simulink model "exp2"  (R2024b)
settings: Solver=VariableStepAuto  StartTime=0.0  StopTime=1  RelTol=1e-3
InitFcn:
  | VOC = 32.9;
  | Iscn = 8.21;
  | k = 1.38e-23;
  | NS = 54;
  | Np = 1;
  | G1 = 1000;
  | G2 = 806;
  | G3 = 506;
  | Gn = 1000;
  | Kv = -0.0123;
  | K1 = 0.0032;
  | T = 301;
  | Tn = 300;
  | q = 1.6e-19;
  | T0n = 9.58e-8;
  | Eg = 1.12;
  | Ign = 8.214;
  | Rs = 0.221;
  | Rp = 414.5;
  | a = 1.0;
libraries: spsVoltageMeasurementLib x7, spsSeriesRLCBranchLib x6, spsDiodeLib x3, spsControlledCurrentSourceLib x3, spsControlledVoltageSourceLib x1, spsCurrentMeasurementLib x1, simulink x1, spspowerguiLib x1
settings Model: Creator=91861  LastModifiedBy=palla

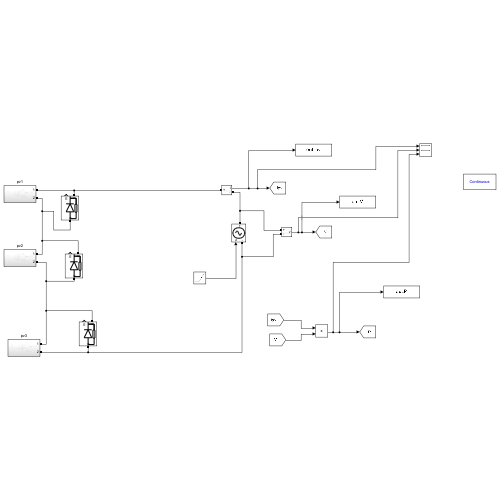
[thumbnail: Simulink's stored preview of the top-level diagram]
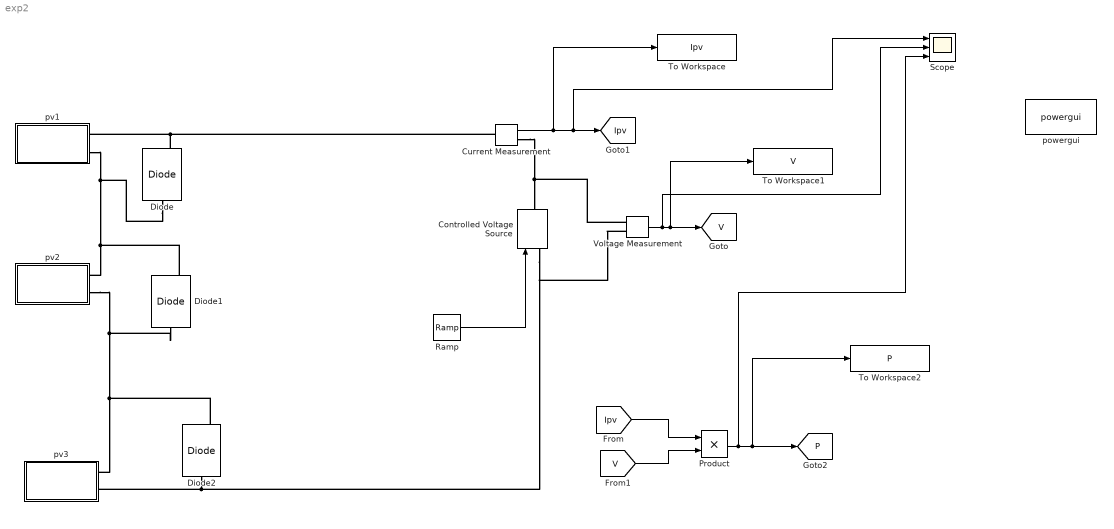
== system exp2 ==
  Controlled Voltage Source : spsControlledVoltageSourceLib/Controlled Voltage Source  Initialize=on  Source_Type=AC  Amplitude=0  Phase=0  Frequency=0  Measurements=None
  Current Measurement : spsCurrentMeasurementLib/Current Measurement  PhasorSimulation=off  OutputType=Complex  PSBequivalent=0
  Diode : spsDiodeLib/Diode  Ron=0.001  Lon=0  Vf=0.8  IC=0  UseSnubber=0  Rs=500  Cs=250e-9  Measurements=on
  Diode1 : spsDiodeLib/Diode  Ron=0.001  Lon=0  Vf=0.8  IC=0  UseSnubber=0  Rs=500  Cs=250e-9  Measurements=on
  Diode2 : spsDiodeLib/Diode  Ron=0.001  Lon=0  Vf=0.8  IC=0  UseSnubber=0  Rs=500  Cs=250e-9  Measurements=on
  Product : Product
  Ramp : simulink/Sources/Ramp  slope=100  start=0  InitialOutput=0
  Scope : Scope  NumInputPorts=3
  To Workspace : ToWorkspace  VariableName=Ipv  SampleTime=-1
  To Workspace1 : ToWorkspace  VariableName=V  SampleTime=-1
  To Workspace2 : ToWorkspace  VariableName=P  SampleTime=-1
  Voltage Measurement : spsVoltageMeasurementLib/Voltage Measurement  PhasorSimulation=off  OutputType=Complex  PSBequivalent=0
  powergui : spspowerguiLib/powergui  Priority=1  SimulationMode=Continuous  SampleTime=50e-6  frequency=60  Iterations=50  frequencyindice=0  Pbase=100e6  ErrMax=1e-4  UnitsV=kV  UnitsW=MW  buscounter=0  FunctionMessages=off  echomessages=off  EnableUseOfTLC=off  CurrentSourceSwitches=off  DisableSnubberDevices=off  DisableRonSwitches=off  DisableVfSwitches=off  DisplayEquations=off  AutomaticDiscreteSolvers=off  SolverType=Tustin/Backward Euler (TBE)  Interpol=off  ExternalGateDelay=off  methode=off  Ts=100  x0status=blocks  SPID=on  SwTol=0  HookPort=off  NonlinearTolerance=1e-4  nMaxIteration=100  ContinueOnMaxIteration=off  RestoreLinks=warning  ResistiveCurrentMeasurement=off  Frange=[0:2:500]  Ylog=off  Xlog=on  ShowGrid=off  save=off  variable=ZData  structure=0  ZoomFFT=off  StartTime=0.0  cycles=1  DisplayStyle=1  fundamental=60  FreqAxis=off  MaxFrequency=1000  frequencyindicesteady=1  RmsSteady=1  display=off
  pv1 : Subsystem
  pv2 : Subsystem
  pv3 : Subsystem
  tag scope: Ipv=global, P=global, V=global
  wires:
  Voltage Measurement/1 -> Scope/2, To Workspace1/1, [V]
  Current Measurement/1 -> To Workspace/1, Scope/1, [Ipv]
  Ramp/1 -> Controlled Voltage Source/1
  [Ipv] -> Product/1
  [V] -> Product/2
  Product/1 -> Scope/3, To Workspace2/1, [P]
  connections:
  pv1/LConn2 -- Diode/LConn1 -- Diode1/RConn1 -- pv2/LConn1
  pv2/LConn2 -- Diode1/LConn1 -- Diode2/RConn1 -- pv3/LConn1
  Diode/RConn1 -- Current Measurement/LConn1 -- pv1/LConn1
  Diode2/LConn1 -- Voltage Measurement/LConn2 -- Controlled Voltage Source/LConn1 -- pv3/LConn2
  Current Measurement/RConn1 -- Voltage Measurement/LConn1 -- Controlled Voltage Source/RConn1

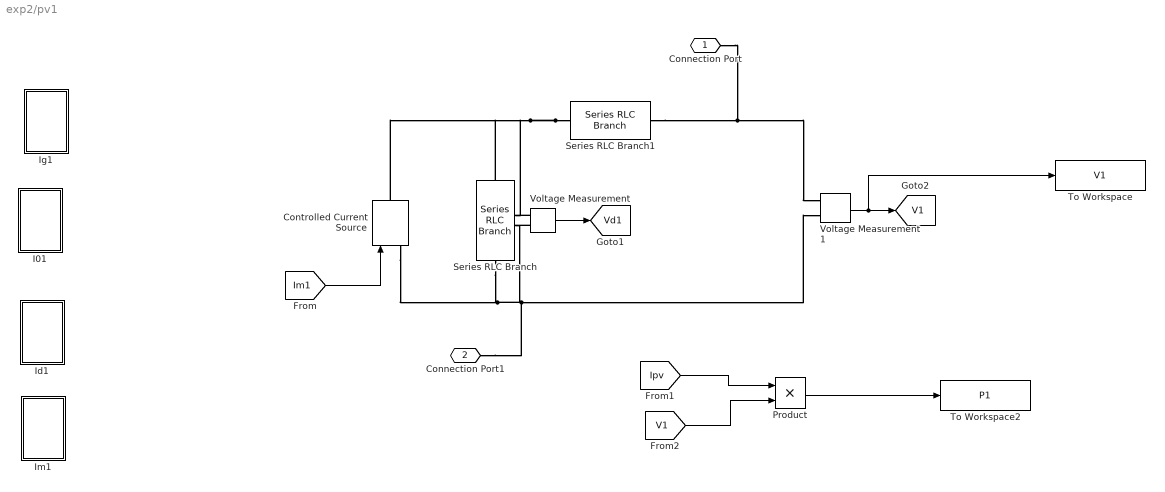
== system exp2/pv1 ==
  Controlled Current Source : spsControlledCurrentSourceLib/Controlled Current Source  Initialize=on  Source_Type=AC  Amplitude=0  Phase=0  Frequency=0  Measurements=None
  I01 : Subsystem
  Id1 : Subsystem
  Ig1 : Subsystem
  Im1 : Subsystem
  Product : Product
  Series RLC Branch : spsSeriesRLCBranchLib/Series RLC Branch  LConnTagsString=__new0  RConnTagsString=__new0  BranchType=R  Resistance=Rp  Inductance=1e-3  SetiL0=off  InitialCurrent=0  Capacitance=1e-6  Setx0=off  InitialVoltage=0  Measurements=None
  Series RLC Branch1 : spsSeriesRLCBranchLib/Series RLC Branch  LConnTagsString=__new0  RConnTagsString=__new0  BranchType=R  Resistance=Rs  Inductance=1e-3  SetiL0=off  InitialCurrent=0  Capacitance=1e-6  Setx0=off  InitialVoltage=0  Measurements=None
  To Workspace : ToWorkspace  VariableName=V1  SampleTime=-1
  To Workspace2 : ToWorkspace  VariableName=P1  SampleTime=-1
  Voltage Measurement : spsVoltageMeasurementLib/Voltage Measurement  PhasorSimulation=off  OutputType=Complex  PSBequivalent=0
  Voltage Measurement1 : spsVoltageMeasurementLib/Voltage Measurement  PhasorSimulation=off  OutputType=Complex  PSBequivalent=0
  Connection Port : PMIOPort  Side=Left
  Connection Port1 : PMIOPort  Port=2  Side=Left
  tag scope: V1=global, Vd1=global
  wires:
  Voltage Measurement1/1 -> To Workspace/1, [V1]
  [Ipv] -> Product/1
  Voltage Measurement/1 -> [Vd1]
  [V1] -> Product/2
  Product/1 -> To Workspace2/1
  [Im1] -> Controlled Current Source/1
  connections:
  Series RLC Branch1/LConn1 -- Controlled Current Source/RConn1 -- Series RLC Branch/LConn1 -- Voltage Measurement/LConn1
  Controlled Current Source/LConn1 -- Series RLC Branch/RConn1 -- Voltage Measurement/LConn2 -- Connection Port1/RConn1 -- Voltage Measurement1/LConn2
  Series RLC Branch1/RConn1 -- Connection Port/RConn1 -- Voltage Measurement1/LConn1

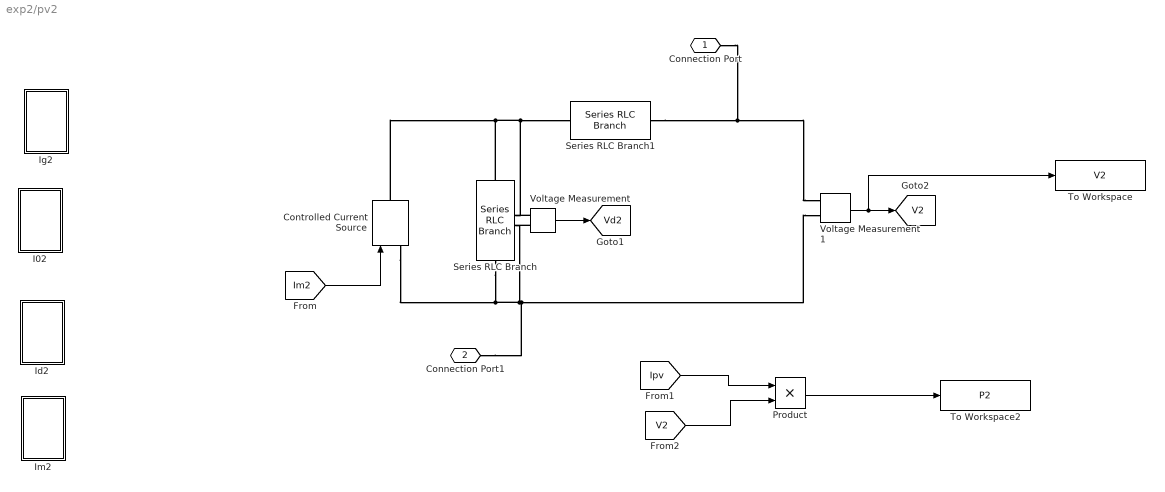
== system exp2/pv2 ==
  Controlled Current Source : spsControlledCurrentSourceLib/Controlled Current Source  Initialize=on  Source_Type=AC  Amplitude=0  Phase=0  Frequency=0  Measurements=None
  I02 : Subsystem
  Id2 : Subsystem
  Ig2 : Subsystem
  Im2 : Subsystem
  Product : Product
  Series RLC Branch : spsSeriesRLCBranchLib/Series RLC Branch  LConnTagsString=__new0  RConnTagsString=__new0  BranchType=R  Resistance=Rp  Inductance=1e-3  SetiL0=off  InitialCurrent=0  Capacitance=1e-6  Setx0=off  InitialVoltage=0  Measurements=None
  Series RLC Branch1 : spsSeriesRLCBranchLib/Series RLC Branch  LConnTagsString=__new0  RConnTagsString=__new0  BranchType=R  Resistance=Rs  Inductance=1e-3  SetiL0=off  InitialCurrent=0  Capacitance=1e-6  Setx0=off  InitialVoltage=0  Measurements=None
  To Workspace : ToWorkspace  VariableName=V2  SampleTime=-1
  To Workspace2 : ToWorkspace  VariableName=P2  SampleTime=-1
  Voltage Measurement : spsVoltageMeasurementLib/Voltage Measurement  PhasorSimulation=off  OutputType=Complex  PSBequivalent=0
  Voltage Measurement1 : spsVoltageMeasurementLib/Voltage Measurement  PhasorSimulation=off  OutputType=Complex  PSBequivalent=0
  Connection Port : PMIOPort  Side=Left
  Connection Port1 : PMIOPort  Port=2  Side=Left
  tag scope: V2=global, Vd2=global
  wires:
  Voltage Measurement1/1 -> To Workspace/1, [V2]
  [Ipv] -> Product/1
  Voltage Measurement/1 -> [Vd2]
  [V2] -> Product/2
  Product/1 -> To Workspace2/1
  [Im2] -> Controlled Current Source/1
  connections:
  Controlled Current Source/RConn1 -- Series RLC Branch/LConn1 -- Voltage Measurement/LConn1 -- Series RLC Branch1/LConn1
  Voltage Measurement1/LConn2 -- Controlled Current Source/LConn1 -- Series RLC Branch/RConn1 -- Voltage Measurement/LConn2 -- Connection Port1/RConn1
  Voltage Measurement1/LConn1 -- Series RLC Branch1/RConn1 -- Connection Port/RConn1

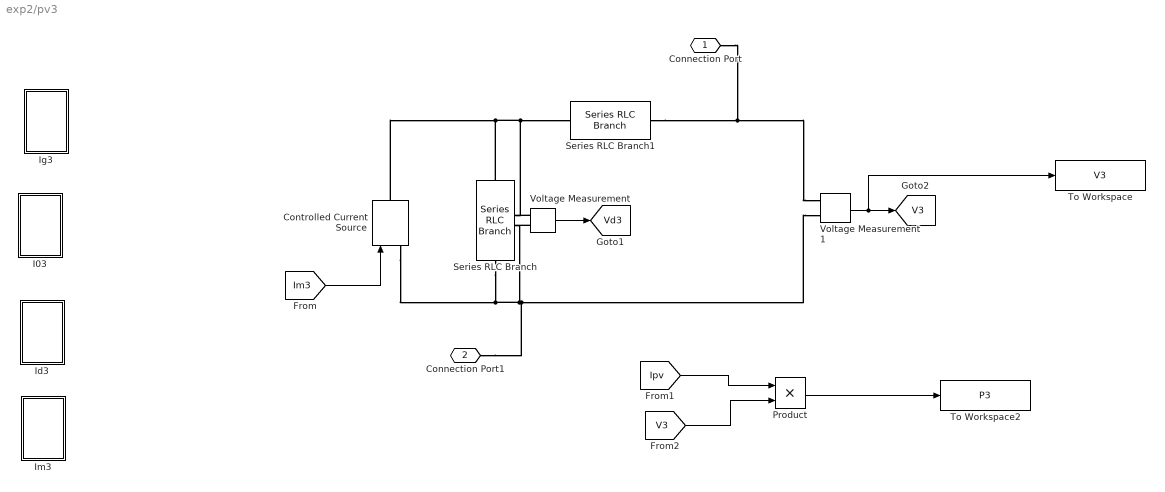
== system exp2/pv3 ==
  Controlled Current Source : spsControlledCurrentSourceLib/Controlled Current Source  Initialize=on  Source_Type=AC  Amplitude=0  Phase=0  Frequency=0  Measurements=None
  I03 : Subsystem
  Id3 : Subsystem
  Ig3 : Subsystem
  Im3 : Subsystem
  Product : Product
  Series RLC Branch : spsSeriesRLCBranchLib/Series RLC Branch  LConnTagsString=__new0  RConnTagsString=__new0  BranchType=R  Resistance=Rp  Inductance=1e-3  SetiL0=off  InitialCurrent=0  Capacitance=1e-6  Setx0=off  InitialVoltage=0  Measurements=None
  Series RLC Branch1 : spsSeriesRLCBranchLib/Series RLC Branch  LConnTagsString=__new0  RConnTagsString=__new0  BranchType=R  Resistance=Rs  Inductance=1e-3  SetiL0=off  InitialCurrent=0  Capacitance=1e-6  Setx0=off  InitialVoltage=0  Measurements=None
  To Workspace : ToWorkspace  VariableName=V3  SampleTime=-1
  To Workspace2 : ToWorkspace  VariableName=P3  SampleTime=-1
  Voltage Measurement : spsVoltageMeasurementLib/Voltage Measurement  PhasorSimulation=off  OutputType=Complex  PSBequivalent=0
  Voltage Measurement1 : spsVoltageMeasurementLib/Voltage Measurement  PhasorSimulation=off  OutputType=Complex  PSBequivalent=0
  Connection Port : PMIOPort  Side=Left
  Connection Port1 : PMIOPort  Port=2  Side=Left
  tag scope: V3=global, Vd3=global
  wires:
  Voltage Measurement1/1 -> To Workspace/1, [V3]
  [Ipv] -> Product/1
  Voltage Measurement/1 -> [Vd3]
  [V3] -> Product/2
  Product/1 -> To Workspace2/1
  [Im3] -> Controlled Current Source/1
  connections:
  Controlled Current Source/RConn1 -- Series RLC Branch/LConn1 -- Voltage Measurement/LConn1 -- Series RLC Branch1/LConn1
  Voltage Measurement1/LConn2 -- Controlled Current Source/LConn1 -- Series RLC Branch/RConn1 -- Voltage Measurement/LConn2 -- Connection Port1/RConn1
  Voltage Measurement1/LConn1 -- Series RLC Branch1/RConn1 -- Connection Port/RConn1

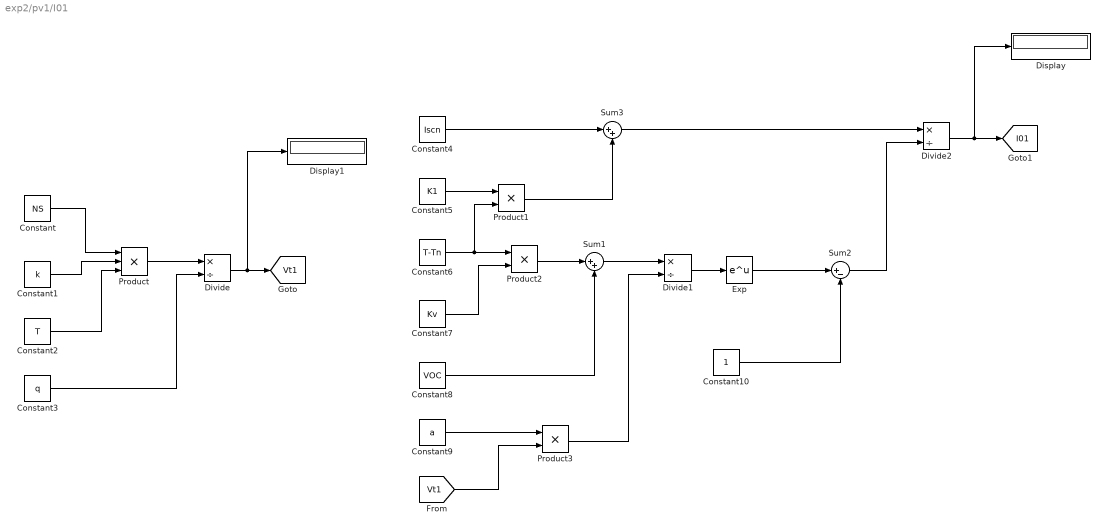
== system exp2/pv1/I01 ==
  Constant : Constant  Value=NS
  Constant1 : Constant  Value=k
  Constant10 : Constant
  Constant2 : Constant  Value=T
  Constant3 : Constant  Value=q
  Constant4 : Constant  Value=Iscn
  Constant5 : Constant  Value=K1
  Constant6 : Constant  Value=T-Tn
  Constant7 : Constant  Value=Kv
  Constant8 : Constant  Value=VOC
  Constant9 : Constant  Value=a
  Display : Display
  Display1 : Display
  Divide : Product  Inputs=*/
  Divide1 : Product  Inputs=*/
  Divide2 : Product  Inputs=*/
  Exp : Math
  Product : Product  Inputs=3
  Product1 : Product
  Product2 : Product
  Product3 : Product
  Sum1 : Sum  Inputs=|++
  Sum2 : Sum  Inputs=|+-
  Sum3 : Sum  Inputs=|++
  tag scope: I01=global, Vt1=global
  wires:
  Constant8/1 -> Sum1/2
  Product2/1 -> Sum1/1
  Constant6/1 -> Product1/2, Product2/1
  Constant5/1 -> Product1/1
  Constant/1 -> Product/1
  Divide2/1 -> Display/1, [I01]
  [Vt1] -> Product3/2
  Product1/1 -> Sum3/2
  Sum1/1 -> Divide1/1
  Sum2/1 -> Divide2/2
  Constant10/1 -> Sum2/2
  Constant7/1 -> Product2/2
  Constant1/1 -> Product/2
  Exp/1 -> Sum2/1
  Product3/1 -> Divide1/2
  Divide/1 -> Display1/1, [Vt1]
  Constant2/1 -> Product/3
  Constant3/1 -> Divide/2
  Divide1/1 -> Exp/1
  Product/1 -> Divide/1
  Constant4/1 -> Sum3/1
  Constant9/1 -> Product3/1
  Sum3/1 -> Divide2/1

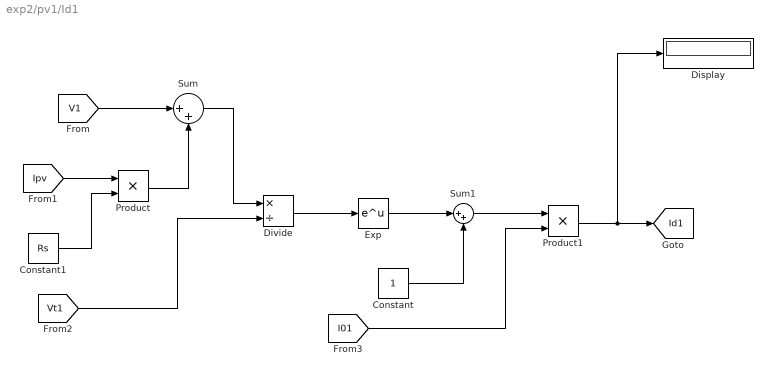
== system exp2/pv1/Id1 ==
  Constant : Constant
  Constant1 : Constant  Value=Rs
  Display : Display
  Divide : Product  Inputs=*/
  Exp : Math
  Product : Product
  Product1 : Product
  Sum : Sum  Inputs=|++
  Sum1 : Sum  Inputs=|++
  tag scope: Id1=global
  wires:
  [Ipv] -> Product/1
  [V1] -> Sum/1
  Divide/1 -> Exp/1
  [Vt1] -> Divide/2
  Sum1/1 -> Product1/1
  Product/1 -> Sum/2
  Constant1/1 -> Product/2
  Product1/1 -> Display/1, [Id1]
  Constant/1 -> Sum1/2
  [I01] -> Product1/2
  Exp/1 -> Sum1/1
  Sum/1 -> Divide/1

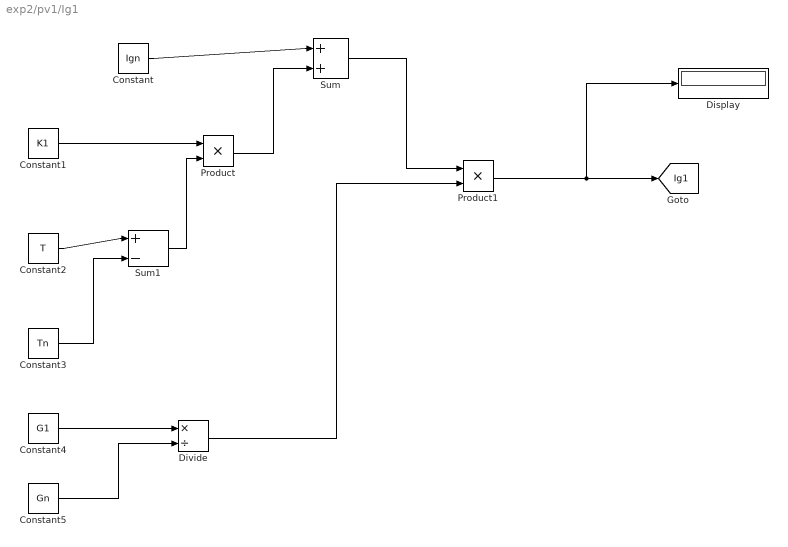
== system exp2/pv1/Ig1 ==
  Constant : Constant  Value=Ign
  Constant1 : Constant  Value=K1
  Constant2 : Constant  Value=T
  Constant3 : Constant  Value=Tn
  Constant4 : Constant  Value=G1
  Constant5 : Constant  Value=Gn
  Display : Display
  Divide : Product  Inputs=*/
  Product : Product
  Product1 : Product
  Sum : Sum  Inputs=|++
  Sum1 : Sum  Inputs=|+-
  tag scope: Ig1=global
  wires:
  Constant2/1 -> Sum1/1
  Sum/1 -> Product1/1
  Constant3/1 -> Sum1/2
  Product1/1 -> [Ig1], Display/1
  Constant/1 -> Sum/1
  Divide/1 -> Product1/2
  Sum1/1 -> Product/2
  Constant4/1 -> Divide/1
  Product/1 -> Sum/2
  Constant5/1 -> Divide/2
  Constant1/1 -> Product/1

== system exp2/pv1/Im1 ==
  Display : Display
  Sum : Sum  Inputs=|+-
  tag scope: Im1=global
  wires:
  Sum/1 -> Display/1, [Im1]
  [Ig1] -> Sum/1
  [Id1] -> Sum/2

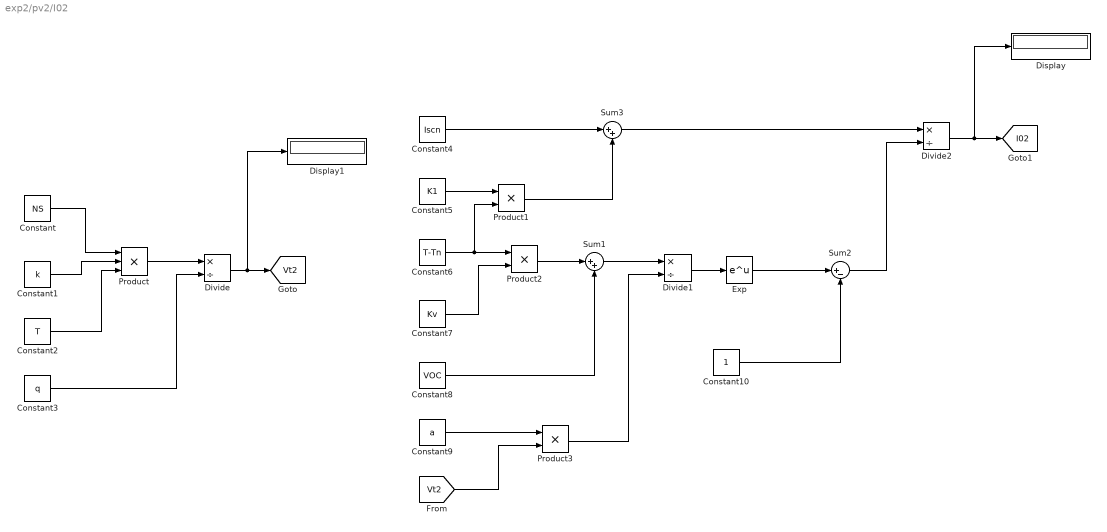
== system exp2/pv2/I02 ==
  Constant : Constant  Value=NS
  Constant1 : Constant  Value=k
  Constant10 : Constant
  Constant2 : Constant  Value=T
  Constant3 : Constant  Value=q
  Constant4 : Constant  Value=Iscn
  Constant5 : Constant  Value=K1
  Constant6 : Constant  Value=T-Tn
  Constant7 : Constant  Value=Kv
  Constant8 : Constant  Value=VOC
  Constant9 : Constant  Value=a
  Display : Display
  Display1 : Display
  Divide : Product  Inputs=*/
  Divide1 : Product  Inputs=*/
  Divide2 : Product  Inputs=*/
  Exp : Math
  Product : Product  Inputs=3
  Product1 : Product
  Product2 : Product
  Product3 : Product
  Sum1 : Sum  Inputs=|++
  Sum2 : Sum  Inputs=|+-
  Sum3 : Sum  Inputs=|++
  tag scope: I02=global, Vt2=global
  wires:
  Constant8/1 -> Sum1/2
  Product2/1 -> Sum1/1
  Constant6/1 -> Product1/2, Product2/1
  Constant5/1 -> Product1/1
  Constant/1 -> Product/1
  Divide2/1 -> Display/1, [I02]
  [Vt2] -> Product3/2
  Product1/1 -> Sum3/2
  Sum1/1 -> Divide1/1
  Sum2/1 -> Divide2/2
  Constant10/1 -> Sum2/2
  Constant7/1 -> Product2/2
  Constant1/1 -> Product/2
  Exp/1 -> Sum2/1
  Product3/1 -> Divide1/2
  Divide/1 -> Display1/1, [Vt2]
  Constant2/1 -> Product/3
  Constant3/1 -> Divide/2
  Divide1/1 -> Exp/1
  Product/1 -> Divide/1
  Constant4/1 -> Sum3/1
  Constant9/1 -> Product3/1
  Sum3/1 -> Divide2/1

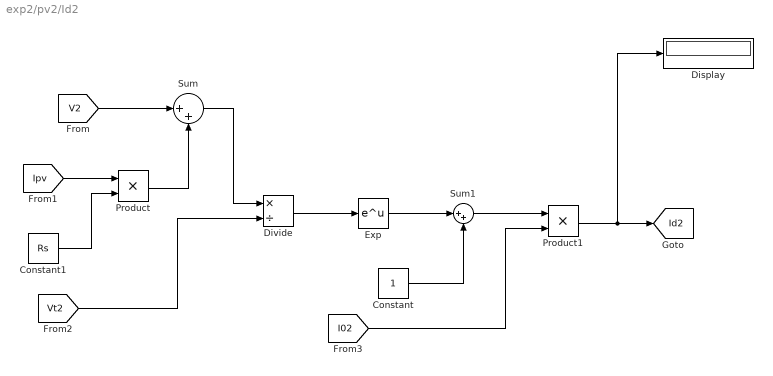
== system exp2/pv2/Id2 ==
  Constant : Constant
  Constant1 : Constant  Value=Rs
  Display : Display
  Divide : Product  Inputs=*/
  Exp : Math
  Product : Product
  Product1 : Product
  Sum : Sum  Inputs=|++
  Sum1 : Sum  Inputs=|++
  tag scope: Id2=global
  wires:
  [Ipv] -> Product/1
  [V2] -> Sum/1
  Divide/1 -> Exp/1
  [Vt2] -> Divide/2
  Sum1/1 -> Product1/1
  Product/1 -> Sum/2
  Constant1/1 -> Product/2
  Product1/1 -> Display/1, [Id2]
  Constant/1 -> Sum1/2
  [I02] -> Product1/2
  Exp/1 -> Sum1/1
  Sum/1 -> Divide/1

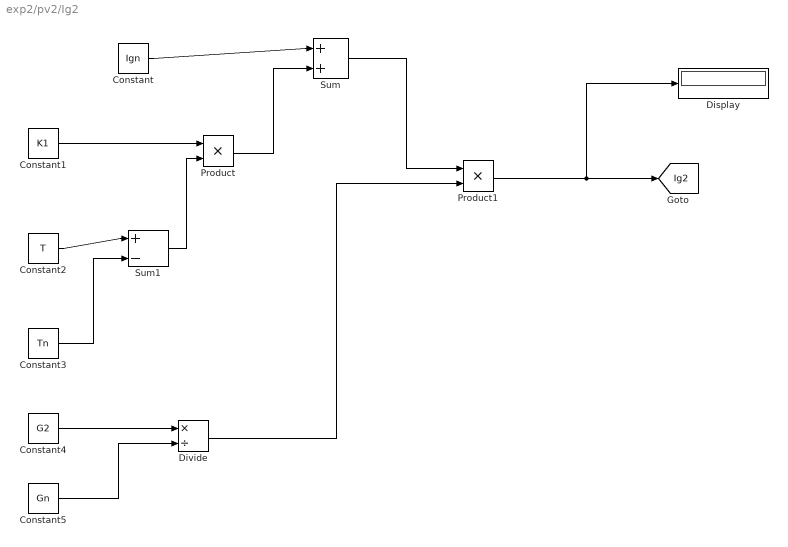
== system exp2/pv2/Ig2 ==
  Constant : Constant  Value=Ign
  Constant1 : Constant  Value=K1
  Constant2 : Constant  Value=T
  Constant3 : Constant  Value=Tn
  Constant4 : Constant  Value=G2
  Constant5 : Constant  Value=Gn
  Display : Display
  Divide : Product  Inputs=*/
  Product : Product
  Product1 : Product
  Sum : Sum  Inputs=|++
  Sum1 : Sum  Inputs=|+-
  tag scope: Ig2=global
  wires:
  Constant2/1 -> Sum1/1
  Sum/1 -> Product1/1
  Constant3/1 -> Sum1/2
  Product1/1 -> [Ig2], Display/1
  Constant/1 -> Sum/1
  Divide/1 -> Product1/2
  Sum1/1 -> Product/2
  Constant4/1 -> Divide/1
  Product/1 -> Sum/2
  Constant5/1 -> Divide/2
  Constant1/1 -> Product/1

== system exp2/pv2/Im2 ==
  Display : Display
  Sum : Sum  Inputs=|+-
  tag scope: Im2=global
  wires:
  Sum/1 -> Display/1, [Im2]
  [Ig2] -> Sum/1
  [Id2] -> Sum/2

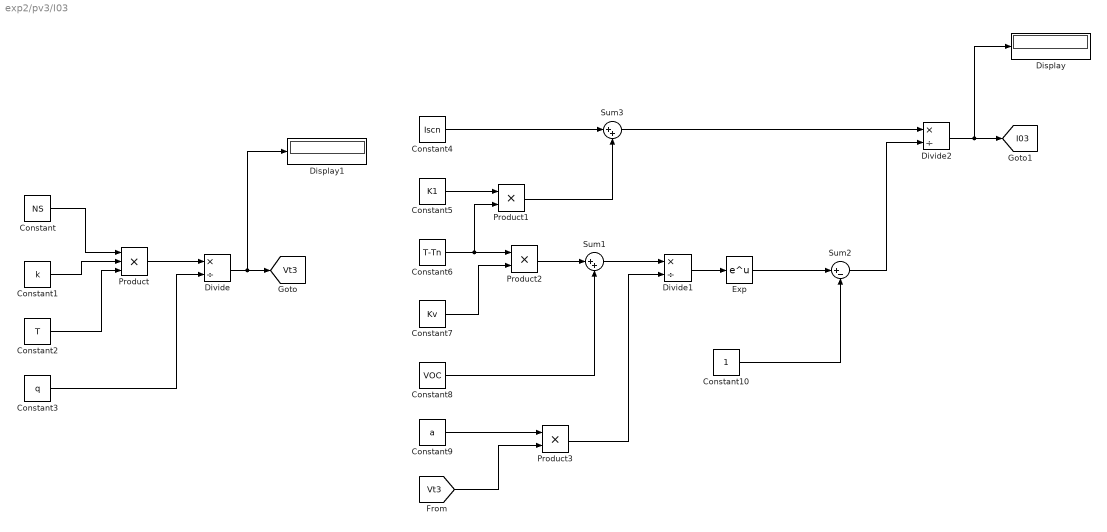
== system exp2/pv3/I03 ==
  Constant : Constant  Value=NS
  Constant1 : Constant  Value=k
  Constant10 : Constant
  Constant2 : Constant  Value=T
  Constant3 : Constant  Value=q
  Constant4 : Constant  Value=Iscn
  Constant5 : Constant  Value=K1
  Constant6 : Constant  Value=T-Tn
  Constant7 : Constant  Value=Kv
  Constant8 : Constant  Value=VOC
  Constant9 : Constant  Value=a
  Display : Display
  Display1 : Display
  Divide : Product  Inputs=*/
  Divide1 : Product  Inputs=*/
  Divide2 : Product  Inputs=*/
  Exp : Math
  Product : Product  Inputs=3
  Product1 : Product
  Product2 : Product
  Product3 : Product
  Sum1 : Sum  Inputs=|++
  Sum2 : Sum  Inputs=|+-
  Sum3 : Sum  Inputs=|++
  tag scope: I03=global, Vt3=global
  wires:
  Constant8/1 -> Sum1/2
  Product2/1 -> Sum1/1
  Constant6/1 -> Product1/2, Product2/1
  Constant5/1 -> Product1/1
  Constant/1 -> Product/1
  Divide2/1 -> Display/1, [I03]
  [Vt3] -> Product3/2
  Product1/1 -> Sum3/2
  Sum1/1 -> Divide1/1
  Sum2/1 -> Divide2/2
  Constant10/1 -> Sum2/2
  Constant7/1 -> Product2/2
  Constant1/1 -> Product/2
  Exp/1 -> Sum2/1
  Product3/1 -> Divide1/2
  Divide/1 -> Display1/1, [Vt3]
  Constant2/1 -> Product/3
  Constant3/1 -> Divide/2
  Divide1/1 -> Exp/1
  Product/1 -> Divide/1
  Constant4/1 -> Sum3/1
  Constant9/1 -> Product3/1
  Sum3/1 -> Divide2/1

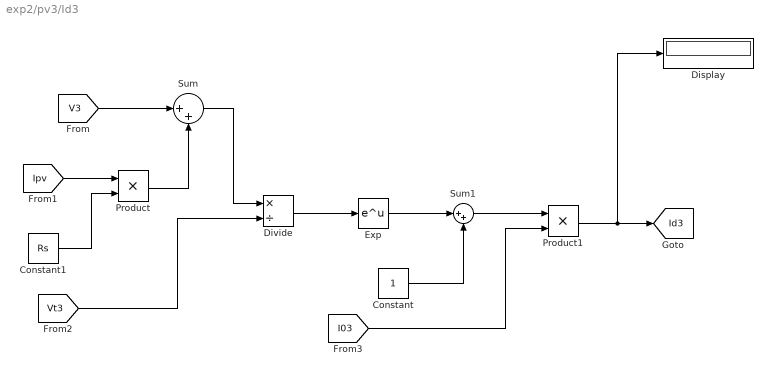
== system exp2/pv3/Id3 ==
  Constant : Constant
  Constant1 : Constant  Value=Rs
  Display : Display
  Divide : Product  Inputs=*/
  Exp : Math
  Product : Product
  Product1 : Product
  Sum : Sum  Inputs=|++
  Sum1 : Sum  Inputs=|++
  tag scope: Id3=global
  wires:
  [Ipv] -> Product/1
  [V3] -> Sum/1
  Divide/1 -> Exp/1
  [Vt3] -> Divide/2
  Sum1/1 -> Product1/1
  Product/1 -> Sum/2
  Constant1/1 -> Product/2
  Product1/1 -> Display/1, [Id3]
  Constant/1 -> Sum1/2
  [I03] -> Product1/2
  Exp/1 -> Sum1/1
  Sum/1 -> Divide/1

== system exp2/pv3/Ig3 ==
  Constant : Constant  Value=Ign
  Constant1 : Constant  Value=K1
  Constant2 : Constant  Value=T
  Constant3 : Constant  Value=Tn
  Constant4 : Constant  Value=G3
  Constant5 : Constant  Value=Gn
  Display : Display
  Divide : Product  Inputs=*/
  Product : Product
  Product1 : Product
  Sum : Sum  Inputs=|++
  Sum1 : Sum  Inputs=|+-
  tag scope: Ig3=global
  wires:
  Constant2/1 -> Sum1/1
  Sum/1 -> Product1/1
  Constant3/1 -> Sum1/2
  Product1/1 -> [Ig3], Display/1
  Constant/1 -> Sum/1
  Divide/1 -> Product1/2
  Sum1/1 -> Product/2
  Constant4/1 -> Divide/1
  Product/1 -> Sum/2
  Constant5/1 -> Divide/2
  Constant1/1 -> Product/1

== system exp2/pv3/Im3 ==
  Display : Display
  Sum : Sum  Inputs=|+-
  tag scope: Im3=global
  wires:
  Sum/1 -> Display/1, [Im3]
  [Ig3] -> Sum/1
  [Id3] -> Sum/2
